simulink model "ModelPreAmp2"  (R2022b)
settings: Solver=FixedStepDiscrete  StartTime=0.0  StopTime=1  RelTol=1e-3  EnableMultiTasking=on
InitFcn:
  | % Initialize model
  | run(['ModelInit.m']);
  | 
  | % load library data
  | GainLibrary_data;
StartFcn:
  | % make sure all the simulated RTC requests are found
  | %RTC_SIM_OBJ.ValidateREQs();
model workspace (MAT data in the model file):
  PreampVolumeTable_Idx = Simulink.Signal
  PreampVolumeTable_Idx.DataType = 'auto'
  PreampVolumeTable_Idx.Dimensions = -1
  PreampVolumeTable_Idx.DimensionsMode = 'auto'
  PreampVolumeTable_Idx.Complexity = 'auto'
  PreampVolumeTable_Idx.SampleTime = -1
  PreampVolumeTable_Idx.SamplingMode = 'auto'
  PreampVolumeTable_Idx.InitialValue = 'uint8([0 255 255 255 255 255])'
  Range = Simulink.Signal
  Range.DataType = 'auto'
  Range.Dimensions = -1
  Range.DimensionsMode = 'auto'
  Range.Complexity = 'auto'
  Range.SampleTime = -1
  Range.SamplingMode = 'auto'
  Table_Idx = Simulink.Signal
  Table_Idx.DataType = 'auto'
  Table_Idx.Dimensions = -1
  Table_Idx.DimensionsMode = 'auto'
  Table_Idx.Complexity = 'auto'
  Table_Idx.SampleTime = -1
  Table_Idx.SamplingMode = 'auto'
undefined symbols (not defined in the file): MedusaConfig, MuteRamper, MuteRamperBtc, numAudioIn, sys_defs
libraries: FeaturePath x12, RTC x5, dspindex x5, SampleRateConverter x4, EdgePorts x2, FadeRamper x2, AudioStats x2, HandyTextFile x2, SleepingBeauty x2, dspsrcs4 x2, Router x1, FadeControl x1
(part 1 of 2)
settings Model: Creator=kl13806  LastModifiedBy=sc48041
settings SolverCC: AlgebraicLoopSolver=TrustRegion  AutoInsertRateTranBlk=on
settings OptimizationCC: DefaultParameterBehavior=Inlined  DefaultUnderspecifiedDataType=single  ZeroExternalMemoryAtStartup=off  ZeroInternalMemoryAtStartup=off  MaxStackSize=2048  DifferentSizesBufferReuse=on  EfficientTunableParamExpr=on
settings DebuggingCC: InheritedTsInSrcMsg=none  MultiTaskDSMMsg=none  MultiTaskRateTransMsg=warning  ParameterPrecisionLossMsg=none  ParameterTunabilityLossMsg=error  UnconnectedInputMsg=warning  UnconnectedOutputMsg=warning  UnconnectedLineMsg=warning  BusObjectLabelMismatch=none  UnknownTsInhSupMsg=none  SFUnexpectedBacktrackingDiag=warning  SFNoUnconditionalDefaultTransitionDiag=warning  SFExecutionAtInitializationDiag=none  SFMachineParentedDataDiag=warning  ArithmeticOperatorsInVariantConditions=warning
settings HardwareCC: ProdBitPerDouble=32  ProdBitPerPointer=32  ProdBitPerSizeT=32  ProdBitPerPtrDiffT=32  ProdLargestAtomicInteger=Long  ProdLargestAtomicFloat=Double  ProdWordSize=32  ProdHWDeviceType=Qualcomm->Hexagon  TargetBitPerPointer=64  TargetBitPerSizeT=64  TargetBitPerPtrDiffT=64  TargetLargestAtomicInteger=Integer  TargetLongLongMode=on  TargetIntDivRoundTo=Zero  TargetEndianess=LittleEndian  TargetWordSize=64  TargetHWDeviceType=MATLAB Host  ProdEqTarget=off
settings ModelReferenceCC: EnableRefExpFcnMdlSchedulingChecks=on
settings SFSimCC: SimUseLocalCustomCode=off  MATLABDynamicMemAlloc=off  CustomCodeUndefinedFunction=UseInterfaceOnly
settings RTWCC: Description=Embedded Coder (host-based shared library target)  SystemTargetFile=ert_shrlib.tlc  GenCodeOnly=on  TemplateMakefile=ert_default_tmf  GenerateReport=on  RetainRTWFile=on  RTWUseLocalCustomCode=off  BuildConfiguration=Faster Runs  IncludeHyperlinkInReport=on  LaunchReport=on  GenerateTraceInfo=on  GenerateTraceReport=on  GenerateTraceReportSl=on  GenerateTraceReportSf=on  GenerateTraceReportEml=on  GenerateCodeMetricsReport=on  GenerateCodeReplacementReport=on
settings CodeAppCC: ForceParamTrailComments=on  IgnoreCustomStorageClasses=off  MaxIdLength=61  OperatorAnnotations=on  SimulinkDataObjDesc=on  SFDataObjDesc=on  MATLABFcnDesc=on  InsertBlockDesc=on  StateflowObjectComments=on  MATLABSourceComments=on
settings STFCustomTargetCC: TargetLangStandard=C99 (ISO)  CodeReplacementLibrary=Qualcomm Hexagon DSP code replacement library  ParMdlRefBuildCompliant=on  CompOptLevelCompliant=on  CombineOutputUpdateFcns=on  ERTCustomFileBanners=on  SupportContinuousTime=off  SupportNonInlinedSFcns=off  RemoveResetFunc=on  SupportVariableSizeSignals=on  MATLABClassNameForMDSCustomization=Simulink.SoftwareTarget.ERTCustomization  ModelStepFunctionPrototypeControlCompliant=on  UseToolchainInfoCompliant=on  SystemTargetFile=ert_shrlib.tlc
settings ERTTargetCC: TargetLangStandard=C99 (ISO)  CodeReplacementLibrary=Qualcomm Hexagon DSP code replacement library  MultiwordLength=2048  ConcurrentExecutionCompliant=off  SupportVariableSizeSignals=on  CPPClassGenCompliant=off  InlinedParameterPlacement=NonHierarchical  ERTCustomFileTemplate=example_file_process.tlc  IndentStyle=Allman  IndentSize=4
settings ConfigComp: CovMetricSettings=dw  CovSaveCumulativeToWorkspaceVar=on  CovSaveSingleToWorkspaceVar=on  CovExternalEMLEnable=off

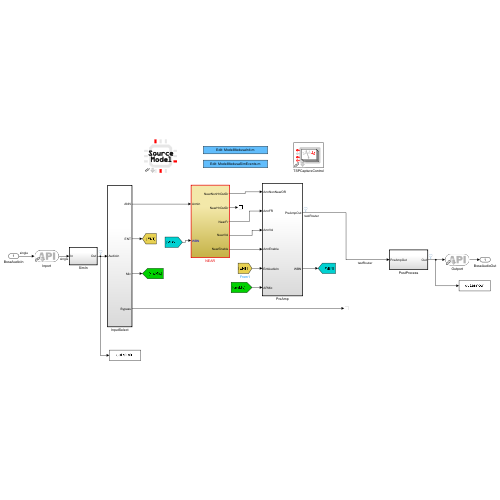
[thumbnail: Simulink's stored preview of the top-level diagram]
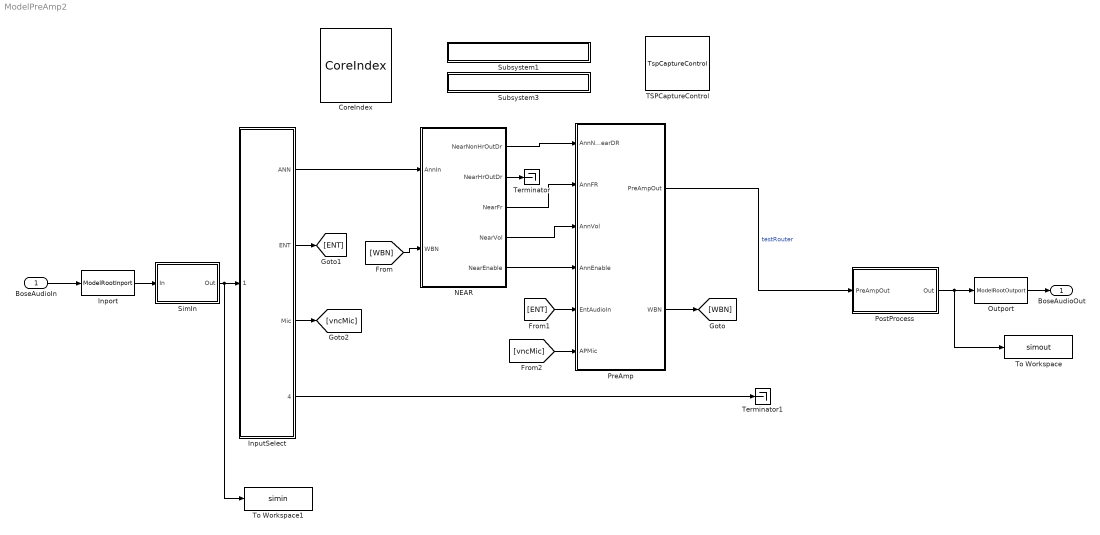
== system ModelPreAmp2 ==
  BoseAudioIn : Inport  OutDataTypeStr=single  PortDimensions=[sys_defs.frameSize numAudioIn]  SampleTime=1/sys_defs.Fs * sys_defs.frameSize
  CoreIndex : FeaturePath/CoreIndex  Role=Source Model  CoreIndex=8  Config=[]  AddressingMode=Directly include core number in message identifiers (i.e. simple and static)  CrossCoreApi=None  CrossCoreAllocation=None  CrossCoreSampleTime=-1  BasePeriod=[]  TriggerInit=[-15 -776 80 -679]
      settings: SourceProductName=Bose Talaria
  Inport : EdgePorts/ModelRootInport  Config=ModelRootIn
      settings: SourceProductName=Bose Talaria
  InputSelect : Subsystem  TreatAsAtomicUnit=on
      settings: RTWSystemCode=Nonreusable function
  NEAR : Subsystem  TreatAsAtomicUnit=on
  Outport : EdgePorts/ModelRootOutport  Config=ModelRootOut
      settings: SourceProductName=Bose Talaria
  PostProcess : Subsystem  TreatAsAtomicUnit=on
  PreAmp : Subsystem  TreatAsAtomicUnit=on
  SimIn : Subsystem  TreatAsAtomicUnit=on
  Subsystem1 : Subsystem  mask{filename=Init.m}
      settings: OpenFcn=edit([ ModelRootName() get(gcbh,'filename') ]);
      mask Display: disp(['Edit: ' ModelRootName() get(gcbh,'filename')]);
  Subsystem3 : Subsystem  mask{filename=SimEvents.m}
      settings: OpenFcn=edit([ ModelRootName() get(gcbh,'filename') ]);
      mask Display: disp(['Edit: ' ModelRootName() get(gcbh,'filename')]);
  TSPCaptureControl : TSP/TspCaptureControl  TriggerInit=[415 -766 500 -694]
      settings: SourceProductName=Bose Talaria
  Terminator : Terminator
  Terminator1 : Terminator
  To Workspace : ToWorkspace  VariableName=simout  SaveFormat=Timeseries  SampleTime=-1
  To Workspace1 : ToWorkspace  VariableName=simin  SaveFormat=Timeseries  SampleTime=-1
  BoseAudioOut : Outport  VectorParamsAs1DForOutWhenUnconnected=off
  wires:
  SimIn/1(Out) -> To Workspace1/1, InputSelect/1(AudioIn)
  BoseAudioIn/1 -> Inport/1
  Inport/1 -> SimIn/1(In)
  Outport/1 -> BoseAudioOut/1
  InputSelect/1(ANN) -> NEAR/1(AnnIn)
  [WBN] -> NEAR/2(WBN)
  NEAR/5(NearEnable) -> PreAmp/4(AnnEnable)
  NEAR/4(NearVol) -> PreAmp/3(AnnVol)
  NEAR/3(NearFr) -> PreAmp/2(AnnFR)
  PreAmp/2(WBN) -> [WBN]
  NEAR/1(NearNonHrOutDr) -> PreAmp/1(AnnNonNearDR)
  InputSelect/2(ENT) -> [ENT]
  [ENT] -> PreAmp/5(EntAudioIn)
  InputSelect/3(Mic) -> [vncMic]
  [vncMic] -> PreAmp/6(APMic)
  PreAmp/1(PreAmpOut) -> PostProcess/1(PreAmpOut)  "testRouter"
  PostProcess/1(Out) -> To Workspace/1, Outport/1
  InputSelect/4(Bypass) -> Terminator1/1
  NEAR/2(NearHrOutDr) -> Terminator/1

== system ModelPreAmp2/InputSelect ==
  AudioIn : Inport
  FeaturePath : FeaturePath/FeaturePath  FeatureName=InputSelect  IsGroup=on  GroupNumber=0  IsModule=on  TriggerInit=[105 216 220 329]
      settings: SourceProductName=Bose Talaria
  Partition : FeaturePath/Partition  PartitionNumber=0  TriggerInit=[250 241 295 309]
      settings: SourceProductName=Bose Talaria
  Reset : Subsystem  Commented=on
  Variable Selector1 : dspindex/Variable Selector  NumInputs=1  rowsOrCols=Columns  IdxMode=Fixed  Elements=entMap  ZerOneIdxMode=One-based  errmode=Clip Index  FillMode=on  FillValues=0
  Variable Selector2 : dspindex/Variable Selector  NumInputs=1  rowsOrCols=Columns  IdxMode=Fixed  Elements=annMap  ZerOneIdxMode=One-based  errmode=Clip Index  FillMode=on  FillValues=0
  Variable Selector3 : dspindex/Variable Selector  NumInputs=1  rowsOrCols=Columns  IdxMode=Fixed  Elements=vncMic  ZerOneIdxMode=One-based  errmode=Clip Index  FillMode=on  FillValues=0
  router : Router/Router  nInRouterMask=inputSelectChanIn  nOutRouterMask=inputSelectChanOut  outputMapDefaultRouterMask=inputSelectOutputMap
  ANN : Outport
  ENT : Outport  Port=2  VectorParamsAs1DForOutWhenUnconnected=off
  Mic : Outport  Port=3
  Bypass : Outport  Port=4  VectorParamsAs1DForOutWhenUnconnected=off
  wires:
  Variable Selector1/1 -> ENT/1
  AudioIn/1 -> Bypass/1, router/1
  router/1 -> Variable Selector3/1, Variable Selector2/1, Variable Selector1/1
  Variable Selector2/1 -> ANN/1
  Variable Selector3/1 -> Mic/1

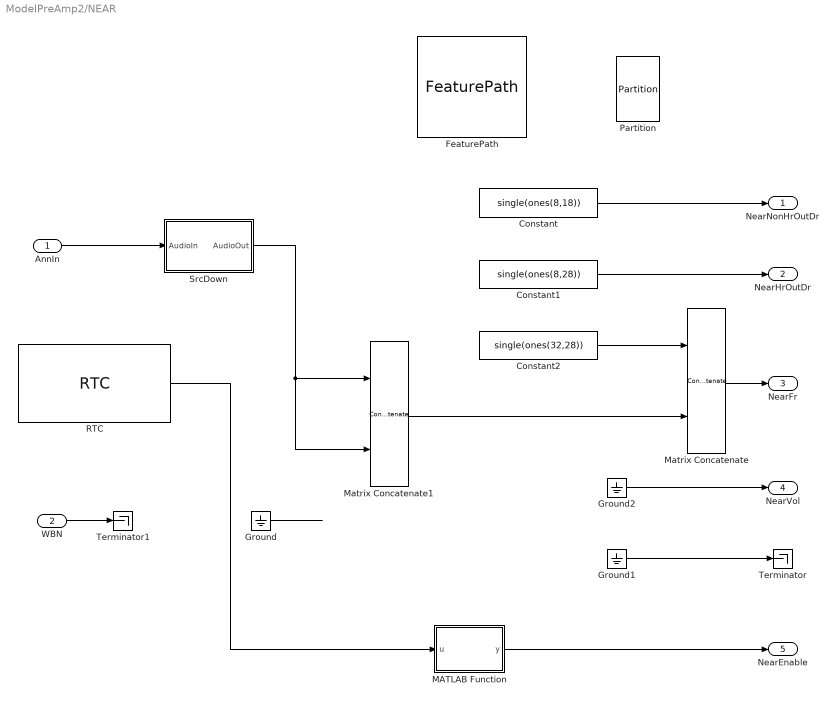
== system ModelPreAmp2/NEAR ==
  AnnIn : Inport
  WBN : Inport  Port=2
  Constant : Constant  Value=single(ones(8,18))
  Constant1 : Constant  Value=single(ones(8,28))
  Constant2 : Constant  Value=single(ones(32,28))
  FeaturePath : FeaturePath/FeaturePath  FeatureName=Near  IsGroup=on  GroupNumber=1  IsModule=on  TriggerInit=[15 -306 130 -199]
      settings: SourceProductName=Bose Talaria
  Ground : Ground
  Ground1 : Ground
  Ground2 : Ground
  MATLAB Function : MATLAB Function  TreatAsAtomicUnit=on
  Matrix Concatenate : Concatenate  Mode=Multidimensional array  ConcatenateDimension=2
  Matrix Concatenate1 : Concatenate  Mode=Multidimensional array  ConcatenateDimension=2
  Partition : FeaturePath/Partition  PartitionNumber=0  TriggerInit=[225 -284 270 -216]
      settings: SourceProductName=Bose Talaria
  RTC : RTC/RTC  REQ_Priority=RTC_Mask.NormalPriority  RequestAtInit=off  EnableRequest=off  REQElemName1=Enable  REQElemType1=uint32  REQElemWidth1=1  REQElemInitial1=[0]  REQElemType2=uint32  REQElemWidth2=1  REQElemInitial2=[]  REQElemType3=uint32  REQElemWidth3=1  REQElemInitial3=[]  REQElemType4=uint32  REQElemWidth4=1  REQElemInitial4=[]  REQElemType5=uint32  REQElemWidth5=1  REQElemInitial5=[]  REQElemType6=uint32  REQElemWidth6=1  REQElemInitial6=[]  REQElemType7=uint32  REQElemWidth7=1  REQElemInitial7=[]  REQElemType8=uint32  REQElemWidth8=1  REQElemInitial8=[]  REQElemType9=uint32  REQElemWidth9=1  REQElemInitial9=[]  REQElemType10=uint32  REQElemWidth10=1  REQElemInitial10=[]  EnableResponse=on  EnableRSP_StatusIn=off  RSPElemType1=uint32  RSPElemWidth1=1  RSPElemType2=uint32  RSPElemWidth2=1  RSPElemType3=uint32  RSPElemWidth3=1  RSPElemType4=uint32  RSPElemWidth4=1  RSPElemType5=uint32  RSPElemWidth5=1  RSPElemType6=uint32  RSPElemWidth6=1  RSPElemType7=uint32  RSPElemWidth7=1  RSPElemType8=uint32  RSPElemWidth8=1  RSPElemType9=uint32  RSPElemWidth9=1  RSPElemType10=uint32  RSPElemWidth10=1  EnableNotification=off  EnableNTF_PrepTrig=off  NTFElemType1=uint32  NTFElemWidth1=1  NTFElemType2=uint32  NTFElemWidth2=1  NTFElemType3=uint32  NTFElemWidth3=1  NTFElemType4=uint32  NTFElemWidth4=1  NTFElemType5=uint32  NTFElemWidth5=1  NTFElemType6=uint32  NTFElemWidth6=1  NTFElemType7=uint32  NTFElemWidth7=1  NTFElemType8=uint32  NTFElemWidth8=1  NTFElemType9=uint32  NTFElemWidth9=1  NTFElemType10=uint32  NTFElemWidth10=1  MaskMessageName=Enable
      settings: SourceProductName=Bose Talaria
  SrcDown : Subsystem  TreatAsAtomicUnit=on
      settings: RTWSystemCode=Nonreusable function
  Terminator : Terminator
  Terminator1 : Terminator
  NearNonHrOutDr : Outport
  NearHrOutDr : Outport  Port=2
  NearFr : Outport  Port=3
  NearVol : Outport  Port=4
  NearEnable : Outport  Port=5
  wires:
  Constant/1 -> NearNonHrOutDr/1
  AnnIn/1 -> SrcDown/1(AudioIn)
  Constant1/1 -> NearHrOutDr/1
  Constant2/1 -> Matrix Concatenate/1
  Matrix Concatenate1/1 -> Matrix Concatenate/2
  Matrix Concatenate/1 -> NearFr/1
  Ground2/1 -> NearVol/1
  Ground1/1 -> Terminator/1
  RTC/1 -> MATLAB Function/1(u)
  MATLAB Function/1(y) -> NearEnable/1
  SrcDown/1(AudioOut) -> Matrix Concatenate1/2, Matrix Concatenate1/1
  Ground/1 -> ?
  WBN/1 -> Terminator1/1

== system ModelPreAmp2/PostProcess ==
  PreAmpOut : Inport
  FeaturePath : FeaturePath/FeaturePath  FeatureName=PostProcess  IsGroup=on  GroupNumber=3  IsModule=on  TriggerInit=[85 -186 200 -79]
      settings: SourceProductName=Bose Talaria
  Matrix Concatenate : Concatenate  Mode=Multidimensional array  ConcatenateDimension=2
  Partition : FeaturePath/Partition  PartitionNumber=0  TriggerInit=[225 -164 270 -96]
      settings: SourceProductName=Bose Talaria
  Reset : Subsystem  Commented=on
  Selector : Selector  NumberOfDimensions=2  InputPortWidth=3  IndexOptions=Select all,Index vector (dialog)  Indices=[1 3],1:2  OutputSizes=1,1
  Out : Outport  VectorParamsAs1DForOutWhenUnconnected=off
  wires:
  PreAmpOut/1 -> Selector/1, Matrix Concatenate/1
  Matrix Concatenate/1 -> Out/1
  Selector/1 -> Matrix Concatenate/2

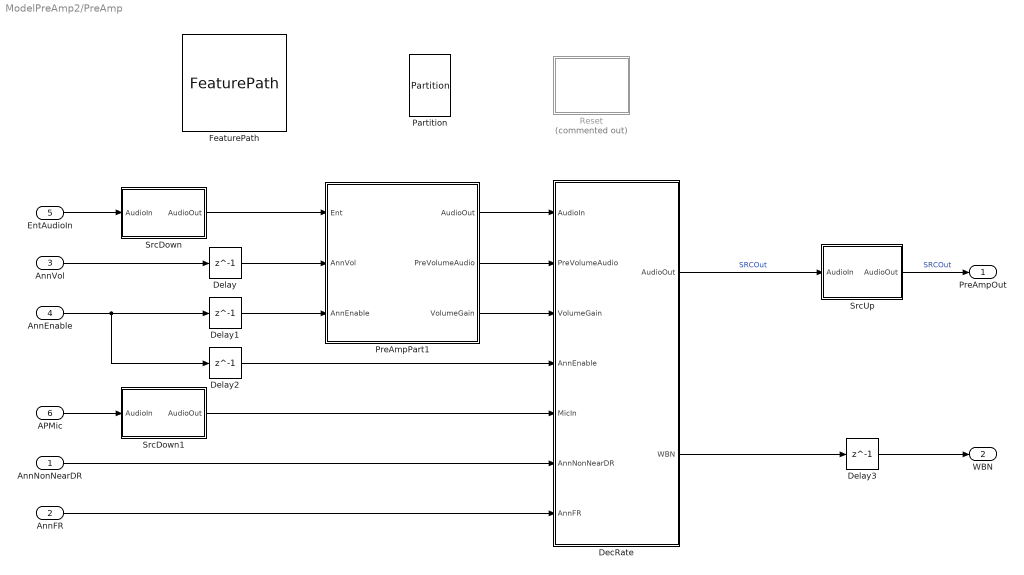
== system ModelPreAmp2/PreAmp ==
  AnnNonNearDR : Inport
  AnnFR : Inport  Port=2
  AnnVol : Inport  Port=3
  AnnEnable : Inport  Port=4
  EntAudioIn : Inport  Port=5
  APMic : Inport  Port=6
  DecRate : Subsystem
  Delay{,1..3} (4 alike) : Delay  DelayLength=1
  FeaturePath : FeaturePath/FeaturePath  FeatureName=PreAmp  IsGroup=on  GroupNumber=2  IsModule=on  TriggerInit=[-135 -246 -20 -139]
      settings: SourceProductName=Bose Talaria
  Partition : FeaturePath/Partition  PartitionNumber=0  TriggerInit=[115 -224 160 -156]
      settings: SourceProductName=Bose Talaria
  PreAmpPart1 : Subsystem  TreatAsAtomicUnit=on
      settings: RTWSystemCode=Nonreusable function
  Reset : Subsystem  Commented=on
  SrcDown : Subsystem  TreatAsAtomicUnit=on
      settings: RTWSystemCode=Nonreusable function
  SrcDown1 : Subsystem  TreatAsAtomicUnit=on
      settings: RTWSystemCode=Nonreusable function
  SrcUp : Subsystem  TreatAsAtomicUnit=on
      settings: RTWSystemCode=Nonreusable function
  PreAmpOut : Outport  VectorParamsAs1DForOutWhenUnconnected=off
  WBN : Outport  Port=2
  wires:
  EntAudioIn/1 -> SrcDown/1(AudioIn)
  DecRate/1(AudioOut) -> SrcUp/1(AudioIn)  "SRCOut"
  SrcUp/1(AudioOut) -> PreAmpOut/1  "SRCOut"
  Delay3/1 -> WBN/1
  SrcDown/1(AudioOut) -> PreAmpPart1/1(Ent)
  AnnVol/1 -> Delay/1
  AnnEnable/1 -> Delay2/1, Delay1/1
  Delay/1 -> PreAmpPart1/2(AnnVol)
  Delay1/1 -> PreAmpPart1/3(AnnEnable)
  AnnNonNearDR/1 -> DecRate/6(AnnNonNearDR)
  AnnFR/1 -> DecRate/7(AnnFR)
  APMic/1 -> SrcDown1/1(AudioIn)
  PreAmpPart1/1(AudioOut) -> DecRate/1(AudioIn)
  PreAmpPart1/2(PreVolumeAudio) -> DecRate/2(PreVolumeAudio)
  PreAmpPart1/3(VolumeGain) -> DecRate/3(VolumeGain)
  Delay2/1 -> DecRate/4(AnnEnable)
  DecRate/2(WBN) -> Delay3/1
  SrcDown1/1(AudioOut) -> DecRate/5(MicIn)

== system ModelPreAmp2/SimIn ==
  In : Inport  OutDataTypeStr=single  SampleTime=1/sys_defs.Fs * sys_defs.frameSize
  Colored Noise : dspsrcs4/Colored Noise  Commented=on  Color=pink  InverseFrequencyPower=1  BoundedOutput=on  NumChannels=2  OutputDataType=single  SamplesPerFrame=32  SampleTime=1/48000  RandomStream=mt19937ar with seed  Seed=67  SimulateUsing=Interpreted execution
  Sine Wave : dspsrcs4/Sine Wave  Amplitude=[0.1*ones(1,numAudioIn)]  Frequency=[150 225 200 275 325]  Phase=zeros(1,numAudioIn)  SampleMode=Discrete  OutComplex=Real  CompMethod=Trigonometric fcn  TableSize=Speed  SampleTime=1/sys_defs.Fs  SamplesPerFrame=sys_defs.frameSize  ResetState=Restart at time zero  OutputFrames=off  dataType=single  wordLen=16  udDataType=sfix(16)  fracBitsMode=Best precision  numFracBits=15  OutDataTypeStr=single  LastOutDataTypeStr=single
  Variant Source : VariantSource  VariantControlMode=sim codegen switching  ShowConditionOnBlock=on
  Out : Outport  VectorParamsAs1DForOutWhenUnconnected=off
  wires:
  In/1 -> Variant Source/2
  Variant Source/1 -> Out/1
  Sine Wave/1 -> Variant Source/1

== system ModelPreAmp2/Subsystem1 ==

== system ModelPreAmp2/Subsystem3 ==

== system ModelPreAmp2/InputSelect/Reset ==
  MATLAB Function : MATLAB Function  TreatAsAtomicUnit=on
  RTC : RTC/RTC  REQ_Priority=RTC_Mask.NormalPriority  RequestAtInit=off  EnableRequest=on  REQElemType1=uint32  REQElemWidth1=1  REQElemInitial1=[]  REQElemType2=uint32  REQElemWidth2=1  REQElemInitial2=[]  REQElemType3=uint32  REQElemWidth3=1  REQElemInitial3=[]  REQElemType4=uint32  REQElemWidth4=1  REQElemInitial4=[]  REQElemType5=uint32  REQElemWidth5=1  REQElemInitial5=[]  REQElemType6=uint32  REQElemWidth6=1  REQElemInitial6=[]  REQElemType7=uint32  REQElemWidth7=1  REQElemInitial7=[]  REQElemType8=uint32  REQElemWidth8=1  REQElemInitial8=[]  REQElemType9=uint32  REQElemWidth9=1  REQElemInitial9=[]  REQElemType10=uint32  REQElemWidth10=1  REQElemInitial10=[]  EnableResponse=on  EnableRSP_StatusIn=off  RSPElemType1=uint32  RSPElemWidth1=1  RSPElemType2=uint32  RSPElemWidth2=1  RSPElemType3=uint32  RSPElemWidth3=1  RSPElemType4=uint32  RSPElemWidth4=1  RSPElemType5=uint32  RSPElemWidth5=1  RSPElemType6=uint32  RSPElemWidth6=1  RSPElemType7=uint32  RSPElemWidth7=1  RSPElemType8=uint32  RSPElemWidth8=1  RSPElemType9=uint32  RSPElemWidth9=1  RSPElemType10=uint32  RSPElemWidth10=1  EnableNotification=off  EnableNTF_PrepTrig=off  NTFElemType1=uint32  NTFElemWidth1=1  NTFElemType2=uint32  NTFElemWidth2=1  NTFElemType3=uint32  NTFElemWidth3=1  NTFElemType4=uint32  NTFElemWidth4=1  NTFElemType5=uint32  NTFElemWidth5=1  NTFElemType6=uint32  NTFElemWidth6=1  NTFElemType7=uint32  NTFElemWidth7=1  NTFElemType8=uint32  NTFElemWidth8=1  NTFElemType9=uint32  NTFElemWidth9=1  NTFElemType10=uint32  NTFElemWidth10=1  MaskMessageName=Reset
      settings: SourceProductName=Bose Talaria
  wires:
  RTC/1 -> MATLAB Function/Trigger

== system ModelPreAmp2/NEAR/SrcDown ==
  AudioIn : Inport
  Frame Conversion1 : FrameConversion  OutFrame=Sample-based
  Frame Conversion2 : FrameConversion
  SampleRateConverter : SampleRateConverter/SampleRateConverter  UPFACTOR=12  DOWNFACTOR=13  OUTFRAME_SIZE=-1  RATE_SELECTOR=Input Sample Rate  FS=48000  FPASSBAND=16500  FHEARING=19000  PASSBAND_RIPPLE=60  STOPBAND_ATTENUATION=60
  AudioOut : Outport
  wires:
  SampleRateConverter/1 -> Frame Conversion1/1
  AudioIn/1 -> Frame Conversion2/1
  Frame Conversion1/1 -> AudioOut/1
  Frame Conversion2/1 -> SampleRateConverter/1

== system ModelPreAmp2/PostProcess/Reset ==
  MATLAB Function : MATLAB Function  TreatAsAtomicUnit=on
  RTC : RTC/RTC  REQ_Priority=RTC_Mask.NormalPriority  RequestAtInit=off  EnableRequest=on  REQElemType1=uint32  REQElemWidth1=1  REQElemInitial1=[]  REQElemType2=uint32  REQElemWidth2=1  REQElemInitial2=[]  REQElemType3=uint32  REQElemWidth3=1  REQElemInitial3=[]  REQElemType4=uint32  REQElemWidth4=1  REQElemInitial4=[]  REQElemType5=uint32  REQElemWidth5=1  REQElemInitial5=[]  REQElemType6=uint32  REQElemWidth6=1  REQElemInitial6=[]  REQElemType7=uint32  REQElemWidth7=1  REQElemInitial7=[]  REQElemType8=uint32  REQElemWidth8=1  REQElemInitial8=[]  REQElemType9=uint32  REQElemWidth9=1  REQElemInitial9=[]  REQElemType10=uint32  REQElemWidth10=1  REQElemInitial10=[]  EnableResponse=on  EnableRSP_StatusIn=off  RSPElemType1=uint32  RSPElemWidth1=1  RSPElemType2=uint32  RSPElemWidth2=1  RSPElemType3=uint32  RSPElemWidth3=1  RSPElemType4=uint32  RSPElemWidth4=1  RSPElemType5=uint32  RSPElemWidth5=1  RSPElemType6=uint32  RSPElemWidth6=1  RSPElemType7=uint32  RSPElemWidth7=1  RSPElemType8=uint32  RSPElemWidth8=1  RSPElemType9=uint32  RSPElemWidth9=1  RSPElemType10=uint32  RSPElemWidth10=1  EnableNotification=off  EnableNTF_PrepTrig=off  NTFElemType1=uint32  NTFElemWidth1=1  NTFElemType2=uint32  NTFElemWidth2=1  NTFElemType3=uint32  NTFElemWidth3=1  NTFElemType4=uint32  NTFElemWidth4=1  NTFElemType5=uint32  NTFElemWidth5=1  NTFElemType6=uint32  NTFElemWidth6=1  NTFElemType7=uint32  NTFElemWidth7=1  NTFElemType8=uint32  NTFElemWidth8=1  NTFElemType9=uint32  NTFElemWidth9=1  NTFElemType10=uint32  NTFElemWidth10=1  MaskMessageName=Reset
      settings: SourceProductName=Bose Talaria
  wires:
  RTC/1 -> MATLAB Function/Trigger

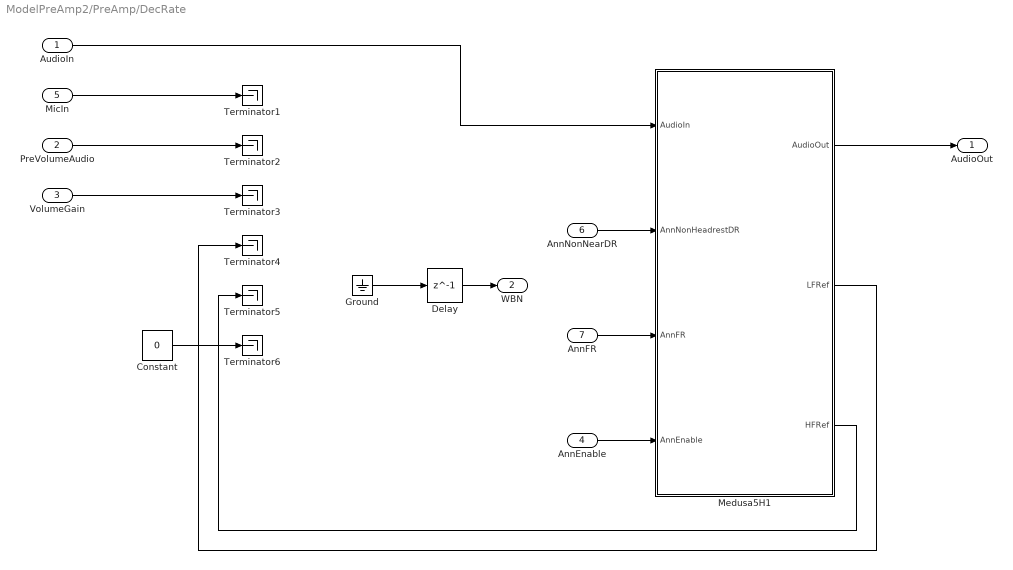
== system ModelPreAmp2/PreAmp/DecRate ==
  AudioIn : Inport
  PreVolumeAudio : Inport  Port=2
  VolumeGain : Inport  Port=3
  AnnEnable : Inport  Port=4
  MicIn : Inport  Port=5
  AnnNonNearDR : Inport  Port=6
  AnnFR : Inport  Port=7
  Constant : Constant  Value=0
  Delay : Delay  DelayLength=1
  Ground : Ground
  Medusa5H1 : Subsystem
  Terminator{1..6} (6 alike) : Terminator
  AudioOut : Outport
  WBN : Outport  Port=2
  wires:
  Medusa5H1/1(AudioOut) -> AudioOut/1
  PreVolumeAudio/1 -> Terminator2/1
  MicIn/1 -> Terminator1/1
  Ground/1 -> Delay/1
  Delay/1 -> WBN/1
  VolumeGain/1 -> Terminator3/1
  Medusa5H1/2(LFRef) -> Terminator4/1
  Medusa5H1/3(HFRef) -> Terminator5/1
  Constant/1 -> Terminator6/1
  AnnEnable/1 -> Medusa5H1/4(AnnEnable)
  AnnNonNearDR/1 -> Medusa5H1/2(AnnNonHeadrestDR)
  AnnFR/1 -> Medusa5H1/3(AnnFR)
  AudioIn/1 -> Medusa5H1/1(AudioIn)

== system ModelPreAmp2/PreAmp/PreAmpPart1 ==
  Ent : Inport
  AnnVol : Inport  Port=2
  AnnEnable : Inport  Port=3
  Delay : Delay  DelayLength=1
  Terminator : Terminator
  Terminator1 : Terminator
  Terminator2 : Terminator
  Volume : VolumeBtc/Volume  FeatureName=Volume  Config=Volume  EnableGainOut=on  TriggerInit=[770 72 845 148]
      settings: SourceProductName=Bose Blocklib
  AudioOut : Outport
  PreVolumeAudio : Outport  Port=2
  VolumeGain : Outport  Port=3
  wires:
  Ent/1 -> Volume/1, PreVolumeAudio/1
  Volume/1 -> AudioOut/1
  Volume/2 -> Delay/1, VolumeGain/1
  AnnVol/1 -> Terminator/1
  AnnEnable/1 -> Terminator1/1
  Delay/1 -> Terminator2/1

== system ModelPreAmp2/PreAmp/Reset ==
  MATLAB Function : MATLAB Function  TreatAsAtomicUnit=on
  RTC : RTC/RTC  REQ_Priority=RTC_Mask.NormalPriority  RequestAtInit=off  EnableRequest=on  REQElemType1=uint32  REQElemWidth1=1  REQElemInitial1=[]  REQElemType2=uint32  REQElemWidth2=1  REQElemInitial2=[]  REQElemType3=uint32  REQElemWidth3=1  REQElemInitial3=[]  REQElemType4=uint32  REQElemWidth4=1  REQElemInitial4=[]  REQElemType5=uint32  REQElemWidth5=1  REQElemInitial5=[]  REQElemType6=uint32  REQElemWidth6=1  REQElemInitial6=[]  REQElemType7=uint32  REQElemWidth7=1  REQElemInitial7=[]  REQElemType8=uint32  REQElemWidth8=1  REQElemInitial8=[]  REQElemType9=uint32  REQElemWidth9=1  REQElemInitial9=[]  REQElemType10=uint32  REQElemWidth10=1  REQElemInitial10=[]  EnableResponse=on  EnableRSP_StatusIn=off  RSPElemType1=uint32  RSPElemWidth1=1  RSPElemType2=uint32  RSPElemWidth2=1  RSPElemType3=uint32  RSPElemWidth3=1  RSPElemType4=uint32  RSPElemWidth4=1  RSPElemType5=uint32  RSPElemWidth5=1  RSPElemType6=uint32  RSPElemWidth6=1  RSPElemType7=uint32  RSPElemWidth7=1  RSPElemType8=uint32  RSPElemWidth8=1  RSPElemType9=uint32  RSPElemWidth9=1  RSPElemType10=uint32  RSPElemWidth10=1  EnableNotification=off  EnableNTF_PrepTrig=off  NTFElemType1=uint32  NTFElemWidth1=1  NTFElemType2=uint32  NTFElemWidth2=1  NTFElemType3=uint32  NTFElemWidth3=1  NTFElemType4=uint32  NTFElemWidth4=1  NTFElemType5=uint32  NTFElemWidth5=1  NTFElemType6=uint32  NTFElemWidth6=1  NTFElemType7=uint32  NTFElemWidth7=1  NTFElemType8=uint32  NTFElemWidth8=1  NTFElemType9=uint32  NTFElemWidth9=1  NTFElemType10=uint32  NTFElemWidth10=1  MaskMessageName=Reset
      settings: SourceProductName=Bose Talaria
  wires:
  RTC/1 -> MATLAB Function/Trigger

== system ModelPreAmp2/PreAmp/SrcDown ==
  AudioIn : Inport
  Frame Conversion1 : FrameConversion  OutFrame=Sample-based
  Frame Conversion2 : FrameConversion
  SampleRateConverter : SampleRateConverter/SampleRateConverter  UPFACTOR=12  DOWNFACTOR=13  OUTFRAME_SIZE=-1  RATE_SELECTOR=Input Sample Rate  FS=48000  FPASSBAND=16500  FHEARING=19000  PASSBAND_RIPPLE=60  STOPBAND_ATTENUATION=60
  AudioOut : Outport
  wires:
  SampleRateConverter/1 -> Frame Conversion1/1
  AudioIn/1 -> Frame Conversion2/1
  Frame Conversion1/1 -> AudioOut/1
  Frame Conversion2/1 -> SampleRateConverter/1

== system ModelPreAmp2/PreAmp/SrcDown1 ==
  AudioIn : Inport
  Frame Conversion1 : FrameConversion  OutFrame=Sample-based
  Frame Conversion2 : FrameConversion
  SampleRateConverter : SampleRateConverter/SampleRateConverter  UPFACTOR=12  DOWNFACTOR=13  OUTFRAME_SIZE=-1  RATE_SELECTOR=Input Sample Rate  FS=48000  FPASSBAND=16500  FHEARING=19000  PASSBAND_RIPPLE=60  STOPBAND_ATTENUATION=60
  AudioOut : Outport
  wires:
  SampleRateConverter/1 -> Frame Conversion1/1
  AudioIn/1 -> Frame Conversion2/1
  Frame Conversion1/1 -> AudioOut/1
  Frame Conversion2/1 -> SampleRateConverter/1

== system ModelPreAmp2/PreAmp/SrcUp ==
  AudioIn : Inport
  Frame Conversion : FrameConversion
  Frame Conversion1 : FrameConversion  OutFrame=Sample-based
  SampleRateConverter1 : SampleRateConverter/SampleRateConverter  UPFACTOR=13  DOWNFACTOR=12  OUTFRAME_SIZE=-1  RATE_SELECTOR=Input Sample Rate  FS=48000  FPASSBAND=16500  FHEARING=19000  PASSBAND_RIPPLE=60  STOPBAND_ATTENUATION=60
  AudioOut : Outport
  wires:
  SampleRateConverter1/1 -> Frame Conversion1/1
  Frame Conversion/1 -> SampleRateConverter1/1
  Frame Conversion1/1 -> AudioOut/1
  AudioIn/1 -> Frame Conversion/1

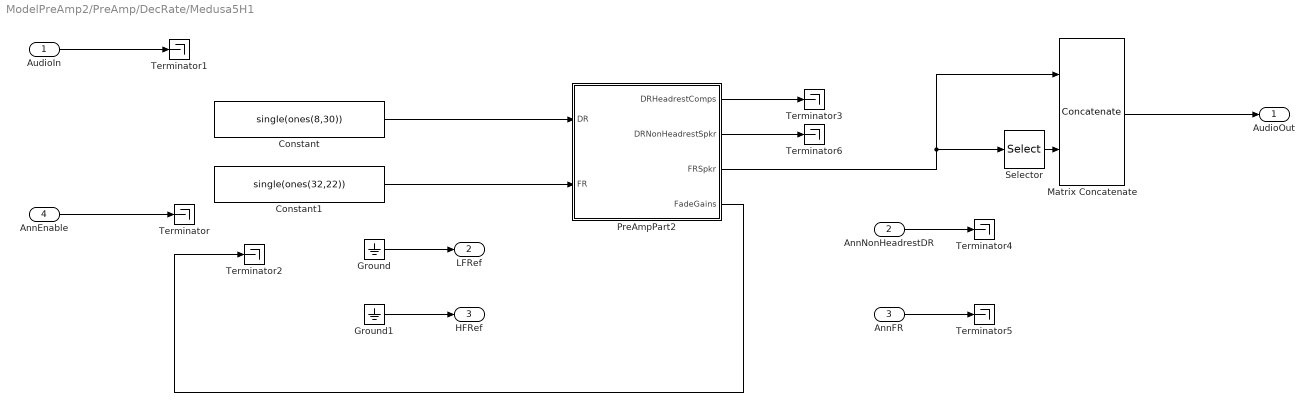
== system ModelPreAmp2/PreAmp/DecRate/Medusa5H1 ==
  AudioIn : Inport
  AnnNonHeadrestDR : Inport  Port=2
  AnnFR : Inport  Port=3
  AnnEnable : Inport  Port=4
  Constant : Constant  Value=single(ones(8,30))
  Constant1 : Constant  Value=single(ones(32,22))
  Ground : Ground
  Ground1 : Ground
  Matrix Concatenate : Concatenate  Mode=Multidimensional array  ConcatenateDimension=2
  PreAmpPart2 : Subsystem
  Selector : Selector  NumberOfDimensions=2  InputPortWidth=3  IndexOptions=Select all,Index vector (dialog)  Indices=[1 3],1:2  OutputSizes=1,1
  Terminator{,1..6} (7 alike) : Terminator
  AudioOut : Outport
  LFRef : Outport  Port=2
  HFRef : Outport  Port=3
  wires:
  Ground1/1 -> HFRef/1
  Ground/1 -> LFRef/1
  AudioIn/1 -> Terminator1/1
  AnnEnable/1 -> Terminator/1
  Constant/1 -> PreAmpPart2/1(DR)
  Constant1/1 -> PreAmpPart2/2(FR)
  PreAmpPart2/1(DRHeadrestComps) -> Terminator3/1
  PreAmpPart2/4(FadeGains) -> Terminator2/1
  AnnNonHeadrestDR/1 -> Terminator4/1
  AnnFR/1 -> Terminator5/1
  Matrix Concatenate/1 -> AudioOut/1
  PreAmpPart2/3(FRSpkr) -> Selector/1, Matrix Concatenate/1
  Selector/1 -> Matrix Concatenate/2
  PreAmpPart2/2(DRNonHeadrestSpkr) -> Terminator6/1

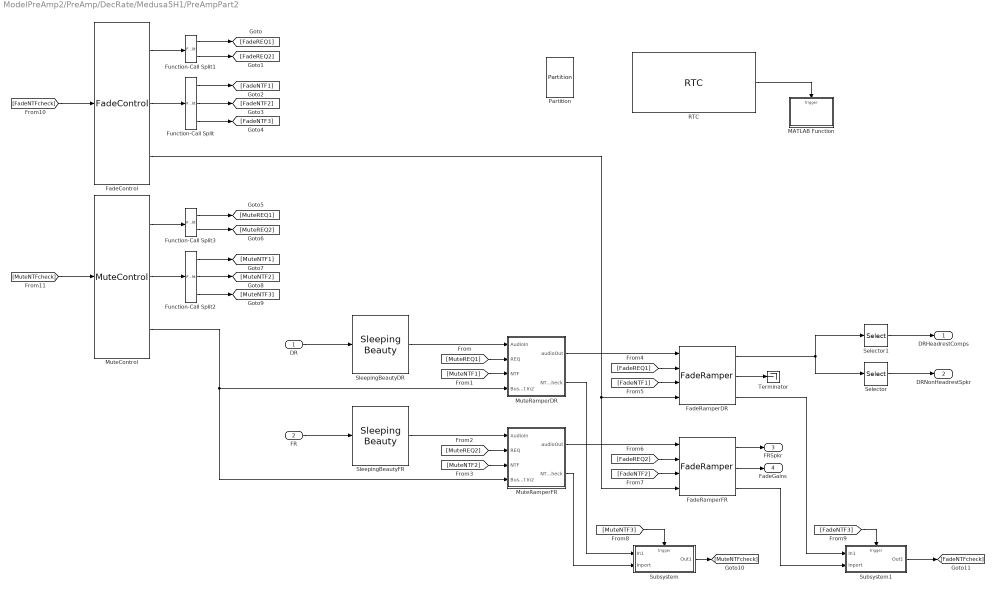
== system ModelPreAmp2/PreAmp/DecRate/Medusa5H1/PreAmpPart2 ==
  DR : Inport
  FR : Inport  Port=2
  FadeControl : FadeControl/FadeControl  BankNumber=0  MaskIndexOffset=128  MaskBoostDisable=off  MaskSilentExtreme=on
  FadeRamperDR : FadeRamper/FadeRamper  MaskFeatureName=FadeRamperDR  MaskChanRampMap=ones(1,30)  MaskEnableGainPort=on
  FadeRamperFR : FadeRamper/FadeRamper  MaskFeatureName=FadeRamperFR  MaskChanRampMap=ones(1,22)  MaskEnableGainPort=on
  Function-Call Split : FunctionCallSplit  IconShape=distinctive  NumOutputPorts=3  OutputPortLayout=default
  Function-Call Split1 : FunctionCallSplit  IconShape=distinctive  NumOutputPorts=2  OutputPortLayout=default
  Function-Call Split2 : FunctionCallSplit  IconShape=distinctive  NumOutputPorts=3  OutputPortLayout=default
  Function-Call Split3 : FunctionCallSplit  IconShape=distinctive  NumOutputPorts=2  OutputPortLayout=default
  MATLAB Function : MATLAB Function  TreatAsAtomicUnit=on
  MuteControl : MuteControl/MuteControl
  MuteRamperDR : Subsystem  AncestorBlock=MuteRamper/MuteRamper  mask(Bose MuteRamper){initial_mute_state=0, samplesPerFrame=8}
      mask prompts: initial_mute_state "Initially muted (logical)"; samplesPerFrame "Samples per Frame"
      mask help: This component is to be used in conjunction with the MuteControl block, which provides runtime control and tuning capabilities via an RTC and the tune variable muteControlRampTime. Multiple instances of this block may be placed within an audio application, and a single MuteControl block has the ability to control all of these rampers simultaneously.
      mask init:
      | blkh = gcbh;
      | % Copy discrete mask parameters into a classdef object
      | InnerLinkConfig = MuteRamperConfig;
      | InnerLinkConfig.InitialMuteState = initial_mute_state;
      | InnerLinkConfig.SamplesPerFrame = samplesPerFrame;
      settings: LibrarySourceBlock=MuteRamper/MuteRamper
  MuteRamperFR : Subsystem  AncestorBlock=MuteRamper/MuteRamper  mask(Bose MuteRamper){initial_mute_state=0, samplesPerFrame=32}
      mask prompts: initial_mute_state "Initially muted (logical)"; samplesPerFrame "Samples per Frame"
      mask help: This component is to be used in conjunction with the MuteControl block, which provides runtime control and tuning capabilities via an RTC and the tune variable muteControlRampTime. Multiple instances of this block may be placed within an audio application, and a single MuteControl block has the ability to control all of these rampers simultaneously.
      mask init: same as ModelPreAmp2/PreAmp/DecRate/Medusa5H1/PreAmpPart2/MuteRamperDR
      settings: LibrarySourceBlock=MuteRamper/MuteRamper
  Partition : FeaturePath/Partition  PartitionNumber=1  TriggerInit=[635 -229 680 -161]
      settings: SourceProductName=Bose Talaria
  RTC : RTC/RTC  REQ_Priority=RTC_Mask.NormalPriority  RequestAtInit=off  EnableRequest=on  REQElemType1=uint32  REQElemWidth1=1  REQElemInitial1=[]  REQElemType2=uint32  REQElemWidth2=1  REQElemInitial2=[]  REQElemType3=uint32  REQElemWidth3=1  REQElemInitial3=[]  REQElemType4=uint32  REQElemWidth4=1  REQElemInitial4=[]  REQElemType5=uint32  REQElemWidth5=1  REQElemInitial5=[]  REQElemType6=uint32  REQElemWidth6=1  REQElemInitial6=[]  REQElemType7=uint32  REQElemWidth7=1  REQElemInitial7=[]  REQElemType8=uint32  REQElemWidth8=1  REQElemInitial8=[]  REQElemType9=uint32  REQElemWidth9=1  REQElemInitial9=[]  REQElemType10=uint32  REQElemWidth10=1  REQElemInitial10=[]  EnableResponse=on  EnableRSP_StatusIn=off  RSPElemType1=uint32  RSPElemWidth1=1  RSPElemType2=uint32  RSPElemWidth2=1  RSPElemType3=uint32  RSPElemWidth3=1  RSPElemType4=uint32  RSPElemWidth4=1  RSPElemType5=uint32  RSPElemWidth5=1  RSPElemType6=uint32  RSPElemWidth6=1  RSPElemType7=uint32  RSPElemWidth7=1  RSPElemType8=uint32  RSPElemWidth8=1  RSPElemType9=uint32  RSPElemWidth9=1  RSPElemType10=uint32  RSPElemWidth10=1  EnableNotification=off  EnableNTF_PrepTrig=off  NTFElemType1=uint32  NTFElemWidth1=1  NTFElemType2=uint32  NTFElemWidth2=1  NTFElemType3=uint32  NTFElemWidth3=1  NTFElemType4=uint32  NTFElemWidth4=1  NTFElemType5=uint32  NTFElemWidth5=1  NTFElemType6=uint32  NTFElemWidth6=1  NTFElemType7=uint32  NTFElemWidth7=1  NTFElemType8=uint32  NTFElemWidth8=1  NTFElemType9=uint32  NTFElemWidth9=1  NTFElemType10=uint32  NTFElemWidth10=1  MaskMessageName=ResetSleepingBeauty
      settings: SourceProductName=Bose Talaria
  Selector : Selector  NumberOfDimensions=2  InputPortWidth=3  IndexOptions=Select all,Index vector (dialog)  Indices=[1 3],1:MedusaConfig.numNonHeadrest  OutputSizes=1,1
  Selector1 : Selector  NumberOfDimensions=2  InputPortWidth=3  IndexOptions=Select all,Index vector (dialog)  Indices=[1 3],MedusaConfig.numNonHeadrest+1:MedusaConfig.numDRChan  OutputSizes=1,1
  SleepingBeautyDR : SleepingBeauty/Sleeping Beauty  MaskFeatureName=SleepingBeautyDR  MaskChanRampMap=ones(1,30)  MaskOffset=128  MaskSilentExtremeMutesBass=off
  SleepingBeautyFR : SleepingBeauty/Sleeping Beauty  MaskFeatureName=SleepingBeautyFR  MaskChanRampMap=ones(1,22)  MaskOffset=128  MaskSilentExtremeMutesBass=off
  Subsystem : Subsystem
  Subsystem1 : Subsystem
  Terminator : Terminator
  DRHeadrestComps : Outport
  DRNonHeadrestSpkr : Outport  Port=2
  FRSpkr : Outport  Port=3
  FadeGains : Outport  Port=4
  wires:
  Function-Call Split2/3 -> [MuteNTF3]
  [FadeNTF1] -> FadeRamperDR/3
  FR/1 -> SleepingBeautyFR/1
  Function-Call Split2/2 -> [MuteNTF2]
  Function-Call Split3/2 -> [MuteREQ2]
  MuteControl/2 -> Function-Call Split2/1
  [FadeREQ2] -> FadeRamperFR/2
  Function-Call Split1/2 -> [FadeREQ2]
  FadeControl/2 -> Function-Call Split/1
  [FadeNTF3] -> Subsystem1/Trigger
  Function-Call Split1/1 -> [FadeREQ1]
  [MuteREQ2] -> MuteRamperFR/2(REQ)
  [MuteNTF3] -> Subsystem/Trigger
  [MuteNTF1] -> MuteRamperDR/3(NTF)
  [FadeNTF2] -> FadeRamperFR/3
  FadeControl/1 -> Function-Call Split1/1
  [FadeNTFcheck] -> FadeControl/1
  MuteRamperDR/1(audioOut) -> FadeRamperDR/1
  [MuteREQ1] -> MuteRamperDR/2(REQ)
  Function-Call Split2/1 -> [MuteNTF1]
  Function-Call Split3/1 -> [MuteREQ1]
  SleepingBeautyDR/1 -> MuteRamperDR/1(AudioIn)
  RTC/1 -> MATLAB Function/Trigger
  FadeRamperDR/2 -> Terminator/1
  Selector1/1 -> DRHeadrestComps/1
  MuteRamperFR/2(NTF_check) -> Subsystem/2(Inport)
  Selector/1 -> DRNonHeadrestSpkr/1
  Subsystem/1(Out1) -> [MuteNTFcheck]
  [MuteNTFcheck] -> MuteControl/1
  [FadeREQ1] -> FadeRamperDR/2
  [MuteNTF2] -> MuteRamperFR/3(NTF)
  MuteControl/1 -> Function-Call Split3/1
  Function-Call Split/2 -> [FadeNTF2]
  FadeRamperDR/3 -> Subsystem1/1(In1)
  FadeRamperFR/2 -> FadeGains/1
  Subsystem1/1(Out1) -> [FadeNTFcheck]
  FadeRamperFR/3 -> Subsystem1/2(Inport)
  SleepingBeautyFR/1 -> MuteRamperFR/1(AudioIn)
  DR/1 -> SleepingBeautyDR/1
  MuteRamperDR/2(NTF_check) -> Subsystem/1(In1)
  FadeRamperFR/1 -> FRSpkr/1
  Function-Call Split/3 -> [FadeNTF3]
  FadeRamperDR/1 -> Selector1/1, Selector/1
  MuteControl/3 -> MuteRamperFR/4(Bus Element In2), MuteRamperDR/4(Bus Element In2)
  Function-Call Split/1 -> [FadeNTF1]
  MuteRamperFR/1(audioOut) -> FadeRamperFR/1
  FadeControl/3 -> FadeRamperFR/4, FadeRamperDR/4

== system ModelPreAmp2/PreAmp/DecRate/Medusa5H1/PreAmpPart2/MuteRamperDR ==
  AudioIn : Inport
  REQ : Inport  Port=2
  NTF : Inport  Port=3
  Bus Element In2 : Inport  Port=4
  InnerLink : Subsystem  AncestorBlock=MuteRamperBtc/MuteRamper  mask(Blocklib MuteRamper){Config=InnerLinkConfig}
      mask prompts: Config "MuteRamperConfig"
      mask help: This component is to be used in conjunction with the MuteControl block, which provides runtime control and tuning capabilities via an RTC and the tune variable muteControlRampTime. Multiple instances of this block may be placed within an audio application, and a single MuteControl block has the ability to control all of these rampers simultaneously.
      mask init:
      | blkh=gcbh;
      | Config=BTConfig.Assert(blkh,Config);
      | Config.Validate();
      | 
      | % Set boundary conditions
      | rampRateBounds = [5,50000];
      | rampTimeBounds = [1,3000];
      | 
      | % Setup Dsms
      | theDsms = {'currentGain','targetLinearGain','nFrames'};
      | CscUtil.SetupDsmsForStaticInit(blkh,theDsms);
      settings: LibrarySourceBlock=MuteRamperBtc/MuteRamper
  audioOut : Outport
  NTF_check : Outport  Port=2
  wires:
  Bus Element In2/1 -> InnerLink/4(InBus)
  NTF/1 -> InnerLink/3(NTF)
  REQ/1 -> InnerLink/2(REQ)
  AudioIn/1 -> InnerLink/1(AudioIn)
  InnerLink/2(NTF_check) -> NTF_check/1
  InnerLink/1(audioOut) -> audioOut/1

== system ModelPreAmp2/PreAmp/DecRate/Medusa5H1/PreAmpPart2/MuteRamperFR ==
  AudioIn : Inport
  REQ : Inport  Port=2
  NTF : Inport  Port=3
  Bus Element In2 : Inport  Port=4
  InnerLink : Subsystem  AncestorBlock=MuteRamperBtc/MuteRamper  mask(Blocklib MuteRamper){Config=InnerLinkConfig}
      mask prompts: Config "MuteRamperConfig"
      mask help: This component is to be used in conjunction with the MuteControl block, which provides runtime control and tuning capabilities via an RTC and the tune variable muteControlRampTime. Multiple instances of this block may be placed within an audio application, and a single MuteControl block has the ability to control all of these rampers simultaneously.
      mask init: same as ModelPreAmp2/PreAmp/DecRate/Medusa5H1/PreAmpPart2/MuteRamperDR/InnerLink
      settings: LibrarySourceBlock=MuteRamperBtc/MuteRamper
  audioOut : Outport
  NTF_check : Outport  Port=2
  wires:
  Bus Element In2/1 -> InnerLink/4(InBus)
  NTF/1 -> InnerLink/3(NTF)
  REQ/1 -> InnerLink/2(REQ)
  AudioIn/1 -> InnerLink/1(AudioIn)
  InnerLink/2(NTF_check) -> NTF_check/1
  InnerLink/1(audioOut) -> audioOut/1

== system ModelPreAmp2/PreAmp/DecRate/Medusa5H1/PreAmpPart2/Subsystem ==
  In1 : Inport
  Inport : Inport  Port=2
  Trigger : TriggerPort  TriggerType=function-call  VariantControl=Variant  PortDimensions=1
  AND : Logic  IconShape=distinctive  AllPortsSameDT=off  OutDataTypeStr=boolean
  Out1 : Outport
  wires:
  In1/1 -> AND/1
  AND/1 -> Out1/1
  Inport/1 -> AND/2

== system ModelPreAmp2/PreAmp/DecRate/Medusa5H1/PreAmpPart2/Subsystem1 ==
  In1 : Inport
  Inport : Inport  Port=2
  Trigger : TriggerPort  TriggerType=function-call  VariantControl=Variant  PortDimensions=1
  AND : Logic  IconShape=distinctive  AllPortsSameDT=off  OutDataTypeStr=boolean
  Out1 : Outport
  wires:
  In1/1 -> AND/1
  AND/1 -> Out1/1
  Inport/1 -> AND/2

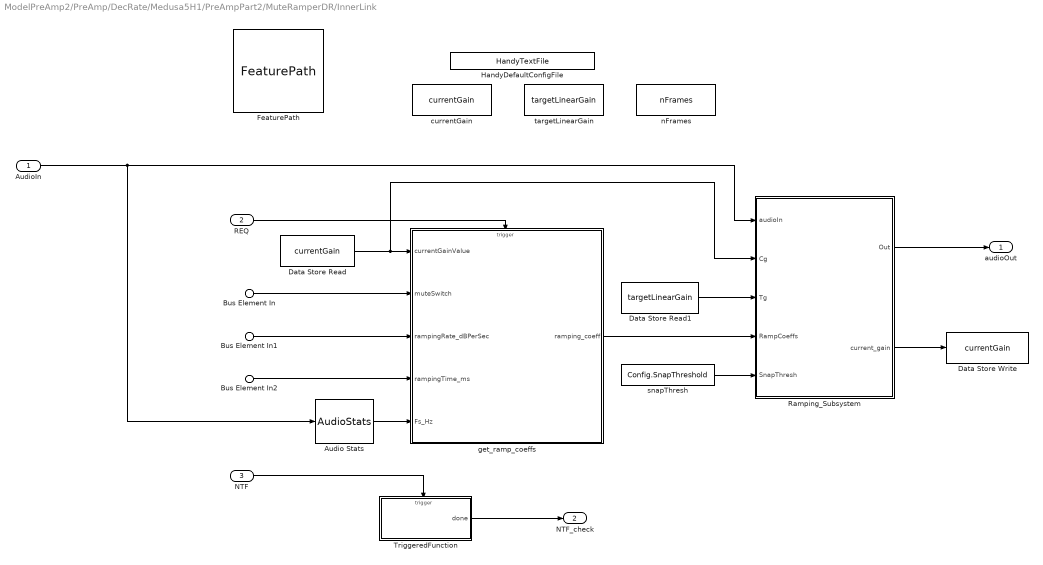
== system ModelPreAmp2/PreAmp/DecRate/Medusa5H1/PreAmpPart2/MuteRamperDR/InnerLink ==
  AudioIn : Inport
  REQ : Inport  Port=2
  NTF : Inport  Port=3
  Bus Element In : Inport  Port=4  PortName=InBus  Element=REQ_mute_switch
  Bus Element In1 : Inport  Port=4  PortName=InBus  Element=rampRate
  Bus Element In2 : Inport  Port=4  PortName=InBus  Element=rampTime
  Audio Stats : AudioStats/AudioStats  DoSampleRate=on  TypeSampleRate=Inherit: auto  DoCallRate=off  TypeCallRate=Inherit: auto  DoFrameSize=off  TypeFrameSize=Inherit: auto  DoChannelCount=off  TypeChannelCount=Inherit: auto  DoTaskRateFactor=off  TypeTaskRateFactor=Inherit: auto  MacroNameRoot=AUDIO  MacroNameRootEval='AUDIO'  IsMacroNameEval=off  MacroSampleRate=off  MacroCallRate=off  MacroFrameSize=off  MacroChannelCount=off  MacroTaskRateFactor=off  MacroTaskId=off  ValidateSampleRate=off  ValueSampleRate=[]  ValidateCallRate=off  ValueCallRate=[]  ValidateFrameSize=off  ValueFrameSize=[]  ValidateChannelCount=off  ValueChannelCount=[]  ValidateTaskRateFactor=off  ValueTaskRateFactor=[]
      settings: SourceProductName=Bose Talaria
  Data Store Read : DataStoreRead  DataStoreName=currentGain  IndexOptions=Index vector (dialog)  Indices=1  OutputSizes=1
  Data Store Read1 : DataStoreRead  DataStoreName=targetLinearGain  IndexOptions=Index vector (dialog)  Indices=1  OutputSizes=1
  Data Store Write : DataStoreWrite  DataStoreName=currentGain  IndexOptions=Index vector (dialog)  Indices=1  OutputSizes=1
  FeaturePath : FeaturePath/FeaturePath  FeatureName=MuteRamperDR  IsGroup=off  GroupNumber=-1  IsModule=off  TriggerInit=[730 -51 845 56]
      settings: SourceProductName=Bose Talaria
  HandyDefaultConfigFile : HandyTextFile/HandyTextFile  TemplateSource=Config  FileSuffix=Init  OpenDialogOnLoad=off  UseThisBlockName=off  AddGrandParentNamePrefix=off  TheDefaultText=|  ShowInLibBrowser=on
      | % $(FILENAME) Setup model parameters for each "Init" callback (e.g. update diagram)
      | sample_rate_in_hertz = 44100;
      | frame_size = 32;
      | sysin_channel_count = 2;
      settings: SourceProductName=Bose Talaria
  Ramping_Subsystem : Subsystem  TreatAsAtomicUnit=on
  TriggeredFunction : MATLAB Function  TreatAsAtomicUnit=on
  currentGain : DataStoreMemory  DataStoreName=currentGain  InitialValue=Config.DlgInitialGainLinear  ShowAdditionalParam=off  OutDataTypeStr=single
  get_ramp_coeffs : MATLAB Function  TreatAsAtomicUnit=on  mask{silentGainLinear=Config.SilentGainLinear, frameSize=Config.SamplesPerFrame}
  nFrames : DataStoreMemory  DataStoreName=nFrames  ShowAdditionalParam=off  OutDataTypeStr=single
  snapThresh : Constant  Value=Config.SnapThreshold  VectorParams1D=off  OutDataTypeStr=single
  targetLinearGain : DataStoreMemory  DataStoreName=targetLinearGain  InitialValue=Config.DlgInitialGainLinear  ShowAdditionalParam=off  OutDataTypeStr=single
  audioOut : Outport  VectorParamsAs1DForOutWhenUnconnected=off
  NTF_check : Outport  Port=2
  wires:
  Data Store Read/1 -> get_ramp_coeffs/1(currentGainValue), Ramping_Subsystem/2(Cg)
  Bus Element In1/1 -> get_ramp_coeffs/3(rampingRate_dBPerSec)
  AudioIn/1 -> Ramping_Subsystem/1(audioIn), Audio Stats/1
  Ramping_Subsystem/1(Out) -> audioOut/1
  get_ramp_coeffs/1(ramping_coeff) -> Ramping_Subsystem/4(RampCoeffs)
  Data Store Read1/1 -> Ramping_Subsystem/3(Tg)
  Bus Element In2/1 -> get_ramp_coeffs/4(rampingTime_ms)
  Ramping_Subsystem/2(current_gain) -> Data Store Write/1
  Bus Element In/1 -> get_ramp_coeffs/2(muteSwitch)
  TriggeredFunction/1(done) -> NTF_check/1
  NTF/1 -> TriggeredFunction/Trigger
  Audio Stats/1 -> get_ramp_coeffs/5(Fs_Hz)
  snapThresh/1 -> Ramping_Subsystem/5(SnapThresh)
  REQ/1 -> get_ramp_coeffs/Trigger

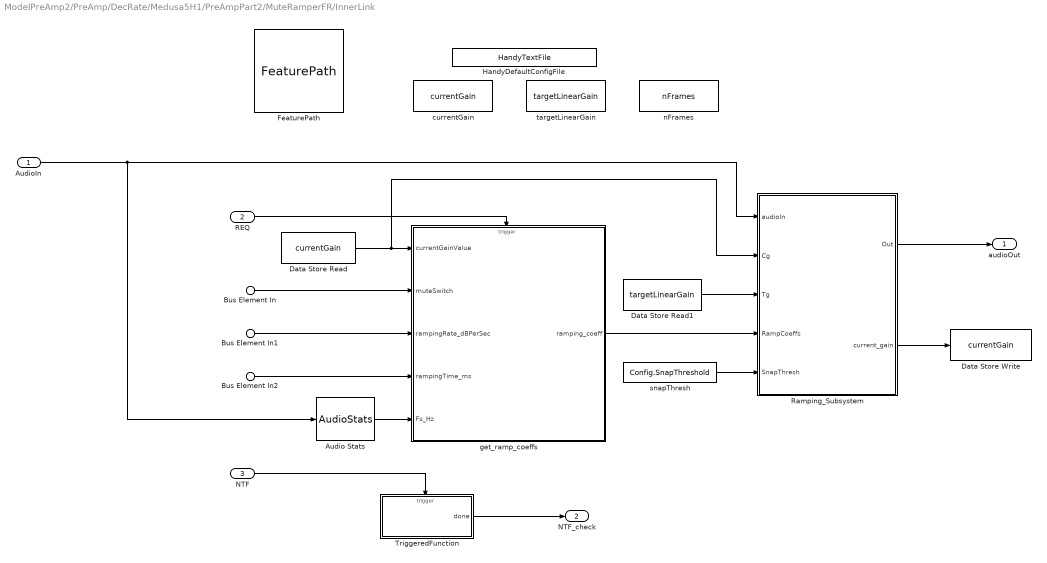
== system ModelPreAmp2/PreAmp/DecRate/Medusa5H1/PreAmpPart2/MuteRamperFR/InnerLink ==
  AudioIn : Inport
  REQ : Inport  Port=2
  NTF : Inport  Port=3
  Bus Element In : Inport  Port=4  PortName=InBus  Element=REQ_mute_switch
  Bus Element In1 : Inport  Port=4  PortName=InBus  Element=rampRate
  Bus Element In2 : Inport  Port=4  PortName=InBus  Element=rampTime
  Audio Stats : AudioStats/AudioStats  DoSampleRate=on  TypeSampleRate=Inherit: auto  DoCallRate=off  TypeCallRate=Inherit: auto  DoFrameSize=off  TypeFrameSize=Inherit: auto  DoChannelCount=off  TypeChannelCount=Inherit: auto  DoTaskRateFactor=off  TypeTaskRateFactor=Inherit: auto  MacroNameRoot=AUDIO  MacroNameRootEval='AUDIO'  IsMacroNameEval=off  MacroSampleRate=off  MacroCallRate=off  MacroFrameSize=off  MacroChannelCount=off  MacroTaskRateFactor=off  MacroTaskId=off  ValidateSampleRate=off  ValueSampleRate=[]  ValidateCallRate=off  ValueCallRate=[]  ValidateFrameSize=off  ValueFrameSize=[]  ValidateChannelCount=off  ValueChannelCount=[]  ValidateTaskRateFactor=off  ValueTaskRateFactor=[]
      settings: SourceProductName=Bose Talaria
  Data Store Read : DataStoreRead  DataStoreName=currentGain  IndexOptions=Index vector (dialog)  Indices=1  OutputSizes=1
  Data Store Read1 : DataStoreRead  DataStoreName=targetLinearGain  IndexOptions=Index vector (dialog)  Indices=1  OutputSizes=1
  Data Store Write : DataStoreWrite  DataStoreName=currentGain  IndexOptions=Index vector (dialog)  Indices=1  OutputSizes=1
  FeaturePath : FeaturePath/FeaturePath  FeatureName=MuteRamperFR  IsGroup=off  GroupNumber=-1  IsModule=off  TriggerInit=[755 -46 870 61]
      settings: SourceProductName=Bose Talaria
  HandyDefaultConfigFile : HandyTextFile/HandyTextFile  TemplateSource=Config  FileSuffix=Init  OpenDialogOnLoad=off  UseThisBlockName=off  AddGrandParentNamePrefix=off  TheDefaultText=|  ShowInLibBrowser=on
      | % $(FILENAME) Setup model parameters for each "Init" callback (e.g. update diagram)
      | sample_rate_in_hertz = 44100;
      | frame_size = 32;
      | sysin_channel_count = 2;
      settings: SourceProductName=Bose Talaria
  Ramping_Subsystem : Subsystem  TreatAsAtomicUnit=on
  TriggeredFunction : MATLAB Function  TreatAsAtomicUnit=on
  currentGain : DataStoreMemory  DataStoreName=currentGain  InitialValue=Config.DlgInitialGainLinear  ShowAdditionalParam=off  OutDataTypeStr=single
  get_ramp_coeffs : MATLAB Function  TreatAsAtomicUnit=on  mask{silentGainLinear=Config.SilentGainLinear, frameSize=Config.SamplesPerFrame}
  nFrames : DataStoreMemory  DataStoreName=nFrames  ShowAdditionalParam=off  OutDataTypeStr=single
  snapThresh : Constant  Value=Config.SnapThreshold  VectorParams1D=off  OutDataTypeStr=single
  targetLinearGain : DataStoreMemory  DataStoreName=targetLinearGain  InitialValue=Config.DlgInitialGainLinear  ShowAdditionalParam=off  OutDataTypeStr=single
  audioOut : Outport  VectorParamsAs1DForOutWhenUnconnected=off
  NTF_check : Outport  Port=2
  wires:
  Data Store Read/1 -> get_ramp_coeffs/1(currentGainValue), Ramping_Subsystem/2(Cg)
  Bus Element In1/1 -> get_ramp_coeffs/3(rampingRate_dBPerSec)
  AudioIn/1 -> Ramping_Subsystem/1(audioIn), Audio Stats/1
  Ramping_Subsystem/1(Out) -> audioOut/1
  get_ramp_coeffs/1(ramping_coeff) -> Ramping_Subsystem/4(RampCoeffs)
  Data Store Read1/1 -> Ramping_Subsystem/3(Tg)
  Bus Element In2/1 -> get_ramp_coeffs/4(rampingTime_ms)
  Ramping_Subsystem/2(current_gain) -> Data Store Write/1
  Bus Element In/1 -> get_ramp_coeffs/2(muteSwitch)
  TriggeredFunction/1(done) -> NTF_check/1
  NTF/1 -> TriggeredFunction/Trigger
  Audio Stats/1 -> get_ramp_coeffs/5(Fs_Hz)
  snapThresh/1 -> Ramping_Subsystem/5(SnapThresh)
  REQ/1 -> get_ramp_coeffs/Trigger

== system ModelPreAmp2/PreAmp/DecRate/Medusa5H1/PreAmpPart2/MuteRamperDR/InnerLink/Ramping_Subsystem ==
  audioIn : Inport
  Cg : Inport  Port=2
  Tg : Inport  Port=3
  RampCoeffs : Inport  Port=4
  SnapThresh : Inport  Port=5
  RampingGain : Subsystem
  Variable Selector : dspindex/Variable Selector  NumInputs=1  rowsOrCols=Rows  IdxMode=Fixed  Elements=Config.SamplesPerFrame  ZerOneIdxMode=One-based  errmode=Clip Index  FillMode=on  FillValues=0
  applyGain : Subsystem
  Out : Outport  VectorParamsAs1DForOutWhenUnconnected=off
  current_gain : Outport  Port=2  VectorParamsAs1DForOutWhenUnconnected=off
  wires:
  RampCoeffs/1 -> RampingGain/3(RampCoeffs)
  Tg/1 -> RampingGain/2(TargetGain)
  SnapThresh/1 -> RampingGain/4(SnapThresh)
  Cg/1 -> RampingGain/1(CurrentGain)
  Variable Selector/1 -> current_gain/1
  applyGain/1(Out1) -> Out/1
  audioIn/1 -> applyGain/2(In2)
  RampingGain/1(current_gain_out) -> Variable Selector/1, applyGain/1(In1)

== system ModelPreAmp2/PreAmp/DecRate/Medusa5H1/PreAmpPart2/MuteRamperFR/InnerLink/Ramping_Subsystem ==
  audioIn : Inport
  Cg : Inport  Port=2
  Tg : Inport  Port=3
  RampCoeffs : Inport  Port=4
  SnapThresh : Inport  Port=5
  RampingGain : Subsystem
  Variable Selector : dspindex/Variable Selector  NumInputs=1  rowsOrCols=Rows  IdxMode=Fixed  Elements=Config.SamplesPerFrame  ZerOneIdxMode=One-based  errmode=Clip Index  FillMode=on  FillValues=0
  applyGain : Subsystem
  Out : Outport  VectorParamsAs1DForOutWhenUnconnected=off
  current_gain : Outport  Port=2  VectorParamsAs1DForOutWhenUnconnected=off
  wires:
  RampCoeffs/1 -> RampingGain/3(RampCoeffs)
  Tg/1 -> RampingGain/2(TargetGain)
  SnapThresh/1 -> RampingGain/4(SnapThresh)
  Cg/1 -> RampingGain/1(CurrentGain)
  Variable Selector/1 -> current_gain/1
  applyGain/1(Out1) -> Out/1
  audioIn/1 -> applyGain/2(In2)
  RampingGain/1(current_gain_out) -> Variable Selector/1, applyGain/1(In1)

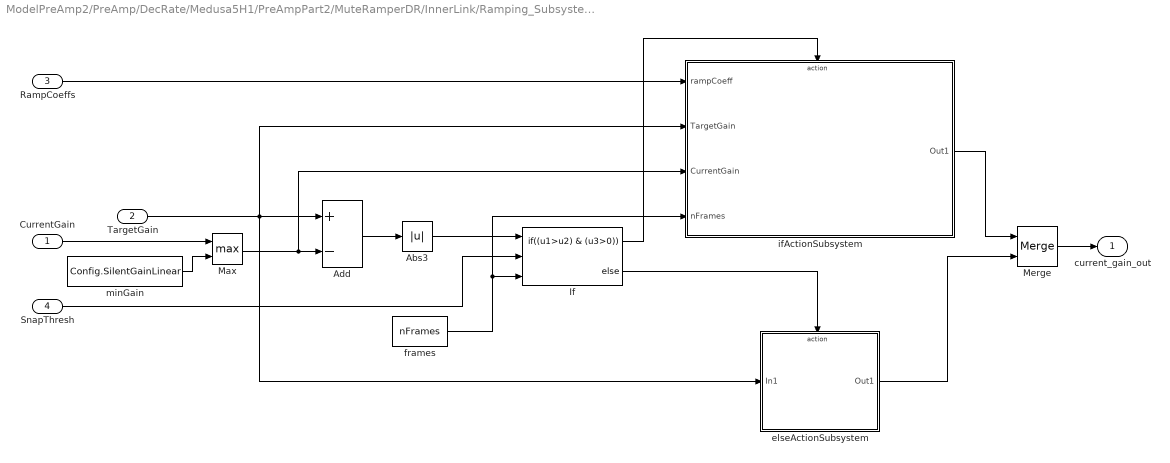
== system ModelPreAmp2/PreAmp/DecRate/Medusa5H1/PreAmpPart2/MuteRamperDR/InnerLink/Ramping_Subsystem/RampingGain ==
  CurrentGain : Inport
  TargetGain : Inport  Port=2
  RampCoeffs : Inport  Port=3
  SnapThresh : Inport  Port=4
  Abs3 : Abs  SaturateOnIntegerOverflow=off
  Add : Sum  Inputs=+-
  If : If  NumInputs=3  IfExpression=(u1>u2) & (u3>0)
  Max : MinMax  Function=max  Inputs=2
  Merge : Merge
  elseActionSubsystem : Subsystem
  frames : DataStoreRead  DataStoreName=nFrames  IndexOptions=Index vector (dialog)  Indices=1  OutputSizes=1
  ifActionSubsystem : Subsystem
  minGain : Constant  Value=Config.SilentGainLinear  OutDataTypeStr=single
  current_gain_out : Outport  VectorParamsAs1DForOutWhenUnconnected=off
  wires:
  frames/1 -> If/3, ifActionSubsystem/4(nFrames)
  elseActionSubsystem/1(Out1) -> Merge/2
  ifActionSubsystem/1(Out1) -> Merge/1
  RampCoeffs/1 -> ifActionSubsystem/1(rampCoeff)
  If/2 -> elseActionSubsystem/Action
  If/1 -> ifActionSubsystem/Action
  CurrentGain/1 -> Max/1
  minGain/1 -> Max/2
  Abs3/1 -> If/1
  SnapThresh/1 -> If/2
  TargetGain/1 -> elseActionSubsystem/1(In1), Add/1, ifActionSubsystem/2(TargetGain)
  Add/1 -> Abs3/1
  Merge/1 -> current_gain_out/1
  Max/1 -> Add/2, ifActionSubsystem/3(CurrentGain)

== system ModelPreAmp2/PreAmp/DecRate/Medusa5H1/PreAmpPart2/MuteRamperDR/InnerLink/Ramping_Subsystem/applyGain ==
  In1 : Inport
  In2 : Inport  Port=2
  For Each Subsystem : Subsystem  TreatAsAtomicUnit=on
  Out1 : Outport  VectorParamsAs1DForOutWhenUnconnected=off
  wires:
  In1/1 -> For Each Subsystem/1(In1)
  For Each Subsystem/1(Out1) -> Out1/1
  In2/1 -> For Each Subsystem/2(In2)

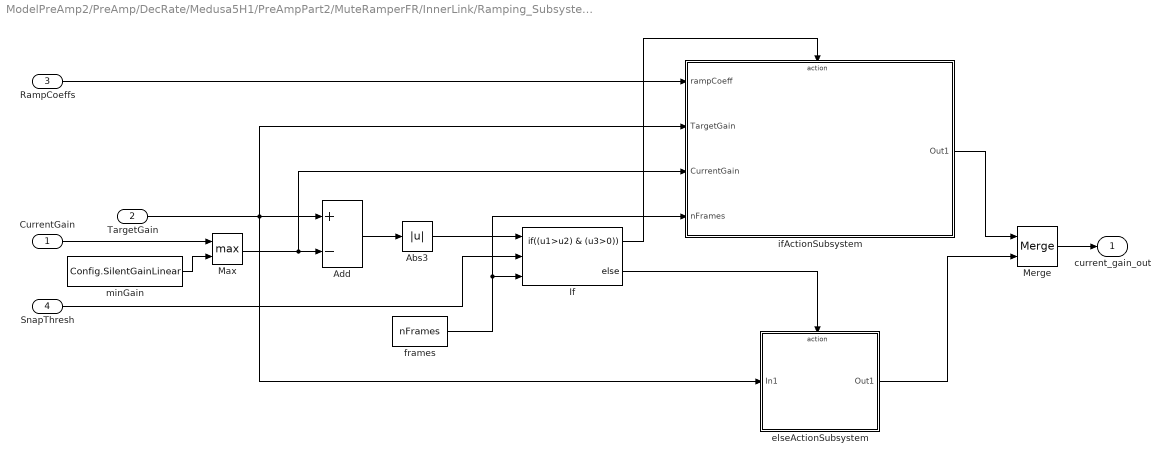
== system ModelPreAmp2/PreAmp/DecRate/Medusa5H1/PreAmpPart2/MuteRamperFR/InnerLink/Ramping_Subsystem/RampingGain ==
  CurrentGain : Inport
  TargetGain : Inport  Port=2
  RampCoeffs : Inport  Port=3
  SnapThresh : Inport  Port=4
  Abs3 : Abs  SaturateOnIntegerOverflow=off
  Add : Sum  Inputs=+-
  If : If  NumInputs=3  IfExpression=(u1>u2) & (u3>0)
  Max : MinMax  Function=max  Inputs=2
  Merge : Merge
  elseActionSubsystem : Subsystem
  frames : DataStoreRead  DataStoreName=nFrames  IndexOptions=Index vector (dialog)  Indices=1  OutputSizes=1
  ifActionSubsystem : Subsystem
  minGain : Constant  Value=Config.SilentGainLinear  OutDataTypeStr=single
  current_gain_out : Outport  VectorParamsAs1DForOutWhenUnconnected=off
  wires:
  frames/1 -> If/3, ifActionSubsystem/4(nFrames)
  elseActionSubsystem/1(Out1) -> Merge/2
  ifActionSubsystem/1(Out1) -> Merge/1
  RampCoeffs/1 -> ifActionSubsystem/1(rampCoeff)
  If/2 -> elseActionSubsystem/Action
  If/1 -> ifActionSubsystem/Action
  CurrentGain/1 -> Max/1
  minGain/1 -> Max/2
  Abs3/1 -> If/1
  SnapThresh/1 -> If/2
  TargetGain/1 -> elseActionSubsystem/1(In1), Add/1, ifActionSubsystem/2(TargetGain)
  Add/1 -> Abs3/1
  Merge/1 -> current_gain_out/1
  Max/1 -> Add/2, ifActionSubsystem/3(CurrentGain)

== system ModelPreAmp2/PreAmp/DecRate/Medusa5H1/PreAmpPart2/MuteRamperFR/InnerLink/Ramping_Subsystem/applyGain ==
  In1 : Inport
  In2 : Inport  Port=2
  For Each Subsystem : Subsystem  TreatAsAtomicUnit=on
  Out1 : Outport  VectorParamsAs1DForOutWhenUnconnected=off
  wires:
  In1/1 -> For Each Subsystem/1(In1)
  For Each Subsystem/1(Out1) -> Out1/1
  In2/1 -> For Each Subsystem/2(In2)

== system ModelPreAmp2/PreAmp/DecRate/Medusa5H1/PreAmpPart2/MuteRamperDR/InnerLink/Ramping_Subsystem/RampingGain/elseActionSubsystem ==
  In1 : Inport
  Action Port : ActionPort  ActionPortLabel=else
  Constant : Constant  Value=ones(Config.SamplesPerFrame,1)  VectorParams1D=off  OutDataTypeStr=single
  Multiply : Product
  Out1 : Outport  VectorParamsAs1DForOutWhenUnconnected=off
  wires:
  Constant/1 -> Multiply/1
  In1/1 -> Multiply/2
  Multiply/1 -> Out1/1
